simulink model "ROS2_simulink_UE5_0821"  (R2024b)
settings: Solver=VariableStepAuto  StartTime=0.0  StopTime=inf  RelTol=1e-3
undefined symbols (not defined in the file): Aw_pont, B_pont, Cb_pont, dt, Earth, I_L, I_T, IC, Ig_CG, k_neg, k_pos, L, l1, l2, LCF, m, rg, Sim3dSensor, T_yaw, trim_setpoint, Umax, WGS84, x, y, z
libraries: sim3dlib x12, ros2lib x8, matrix_library x8, sharedutil x7, uavsimlib x6, simulink x4, simulink_extras x4, sharedtransform x3, robotcorelib x1, aerolibtransform2 x1, sim3dcameralib x1, visionsinks x1
(part 1 of 2)
settings Model: Creator=qwv  LastModifiedBy=qwv

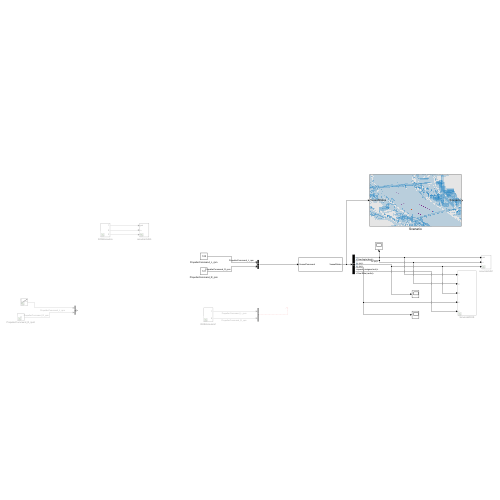
[thumbnail: Simulink's stored preview of the top-level diagram]
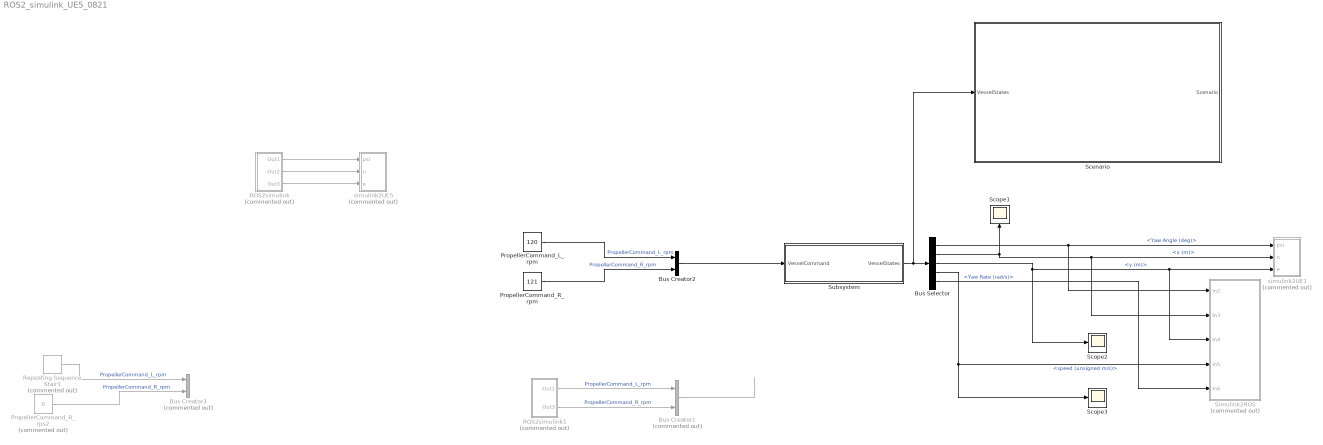
== system ROS2_simulink_UE5_0821 ==
  Bus Creator1 : BusCreator  Commented=on  Inputs=2
  Bus Creator2 : BusCreator  Inputs=3
  Bus Creator3 : BusCreator  Commented=on  Inputs=2
  Bus Selector : BusSelector  OutputSignals=Yaw Angle (deg),x (m),y (m),speed (unsigned m/s),Yaw Rate (rad/s)
  PropellerCommand_L_rpm : Constant  Value=120
  PropellerCommand_R_rpm : Constant  Value=121
  PropellerCommand_R_rps2 : Constant  Commented=on  Value=0
  ROS2simulink : Subsystem  Commented=on
  ROS2simulink1 : Subsystem  Commented=on
  Repeating Sequence Stair1 : simulink/Sources/Repeating Sequence Stair  Commented=on  OutValues=[-320 -300 -280 -260 -240 -220 -200 -180 -160 -140 -120 -100 -80 -60 -40 -20 0 20 40 60 80 100 120 140 160 180 200 220 240 260 280 300 320].'  tsamp=10  OutMin=[]  OutMax=[]  OutDataTypeStr=double  OutputDataTypeScalingMode=double  OutDataType=fixdt(0,8)  ConRadixGroup=Best Precision: Vector-wise  OutScaling=2^-12
  Scenario : Subsystem
      mask Display: image('ScenarioLondon.png'); % Use "Edit Image" on toolstrip to change.
  Scope1 : Scope
  Scope2 : Scope
  Scope3 : Scope
  Simulink2ROS : Subsystem  Commented=on
  Subsystem : Subsystem
  simulink2UE1 : Subsystem  Commented=on
  simulink2UE5 : Subsystem  Commented=on
  wires:
  ROS2simulink/1(Out1) -> simulink2UE5/1(psi)
  ROS2simulink/2(Out2) -> simulink2UE5/2(n)
  ROS2simulink/3(Out3) -> simulink2UE5/3(e)
  Bus Selector/3 -> Simulink2ROS/3(In4), simulink2UE1/3(e), Scope2/1  "<y (m)>"
  Bus Selector/2 -> Simulink2ROS/2(In3), simulink2UE1/2(n), Scope1/1  "<x (m)>"
  Subsystem/1(VesselStates) -> Scenario/1(VesselStates), Bus Selector/1
  Bus Selector/4 -> Scope3/1, Simulink2ROS/4(In5)  "<speed (unsigned m/s)>"
  Bus Selector/1 -> Simulink2ROS/1(In2), simulink2UE1/1(psi)  "<Yaw Angle (deg)>"
  ROS2simulink1/1(Out1) -> Bus Creator1/1  "PropellerCommand_L_rpm"
  ROS2simulink1/2(Out3) -> Bus Creator1/2  "PropellerCommand_R_rpm"
  Bus Selector/5 -> Simulink2ROS/5(In6)  "<Yaw Rate (rad/s)>"
  PropellerCommand_R_rpm/1 -> Bus Creator2/3  "PropellerCommand_R_rpm"
  PropellerCommand_L_rpm/1 -> Bus Creator2/1  "PropellerCommand_L_rpm"
  Bus Creator1/1 -> ?
  Bus Creator2/1 -> Subsystem/1(VesselCommand)
  Repeating Sequence Stair1/1 -> Bus Creator3/1  "PropellerCommand_L_rpm"
  PropellerCommand_R_rps2/1 -> Bus Creator3/2  "PropellerCommand_R_rpm"

== system ROS2_simulink_UE5_0821/ROS2simulink ==
  Blank Message : ros2lib/Blank Message  Commented=on  messageClass=Message  entityType=geometry_msgs/Point  messageType=geometry_msgs/Point  SampleTime=inf
  Bus Assignment : BusAssignment  Commented=on  AssignedSignals=x,z
  Bus Selector : BusSelector  OutputSignals=psi,n,e
  Bus Selector1 : BusSelector  Commented=on  OutputSignals=data
  Constant : Constant  Commented=on
  Constant1 : Constant  Commented=on
  Constant2 : Constant  Commented=on
  Display{,1..3} (4 alike) : Display
  Publish : ros2lib/Publish  Commented=on  topicSource=Specify your own  topic=/my_topic  messageType=geometry_msgs/Twist  QOSHistory=Keep last  QOSDepth=1  QOSReliability=Reliable  QOSDurability=Volatile  QOSDeadline=Inf  QOSLifespan=Inf  QOSLiveliness=Automatic  QOSLeaseDuration=Inf  QOSAvoidROSNamespaceConventions=off
  Sine Wave : Sin  Commented=on  SampleTime=0
  Sine Wave1 : Sin  Commented=on  SampleTime=0
  Subscribe : ros2lib/Subscribe  topicSource=Select from ROS network  topic=/topic_state  messageType=pid_interfaces/Command  sampleTime=-1  QOSHistory=Keep last  QOSDepth=1  QOSReliability=Reliable  QOSDurability=Volatile  QOSDeadline=Inf  QOSLifespan=Inf  QOSLiveliness=Automatic  QOSLeaseDuration=Inf  QOSAvoidROSNamespaceConventions=off
  Out1 : Outport
  Out2 : Outport  Port=2
  Out3 : Outport  Port=3
  wires:
  Bus Assignment/1 -> Publish/1
  Sine Wave1/1 -> Bus Assignment/3
  Blank Message/1 -> Bus Assignment/1
  Sine Wave/1 -> Bus Assignment/2
  Bus Selector/1 -> Out1/1, Display/1  "<psi>"
  Bus Selector/3 -> Out3/1, Display1/1  "<e>"
  Bus Selector/2 -> Display2/1, Out2/1  "<n>"
  Bus Selector1/1 -> Display3/1  "<data>"
  Subscribe/2 -> Bus Selector/1

== system ROS2_simulink_UE5_0821/ROS2simulink1 ==
  Bus Selector : BusSelector  OutputSignals=rpm_e_l,rpm_e_r
  Data Type Conversion : DataTypeConversion  SaturateOnIntegerOverflow=off  RndMeth=Floor
  Data Type Conversion1 : DataTypeConversion  SaturateOnIntegerOverflow=off  RndMeth=Floor
  Display1 : Display
  Display2 : Display
  Subscribe : ros2lib/Subscribe  topicSource=Select from ROS network  topic=/topic_state  messageType=pid_interfaces/Command  sampleTime=-1  QOSHistory=Keep last  QOSDepth=1  QOSReliability=Reliable  QOSDurability=Volatile  QOSDeadline=Inf  QOSLifespan=Inf  QOSLiveliness=Automatic  QOSLeaseDuration=Inf  QOSAvoidROSNamespaceConventions=off
  Out1 : Outport
  Out3 : Outport  Port=2
  wires:
  Bus Selector/2 -> Display1/1, Data Type Conversion1/1  "<rpm_e_r>"
  Subscribe/2 -> Bus Selector/1
  Data Type Conversion/1 -> Out1/1
  Data Type Conversion1/1 -> Out3/1
  Bus Selector/1 -> Data Type Conversion/1, Display2/1  "<rpm_e_l>"

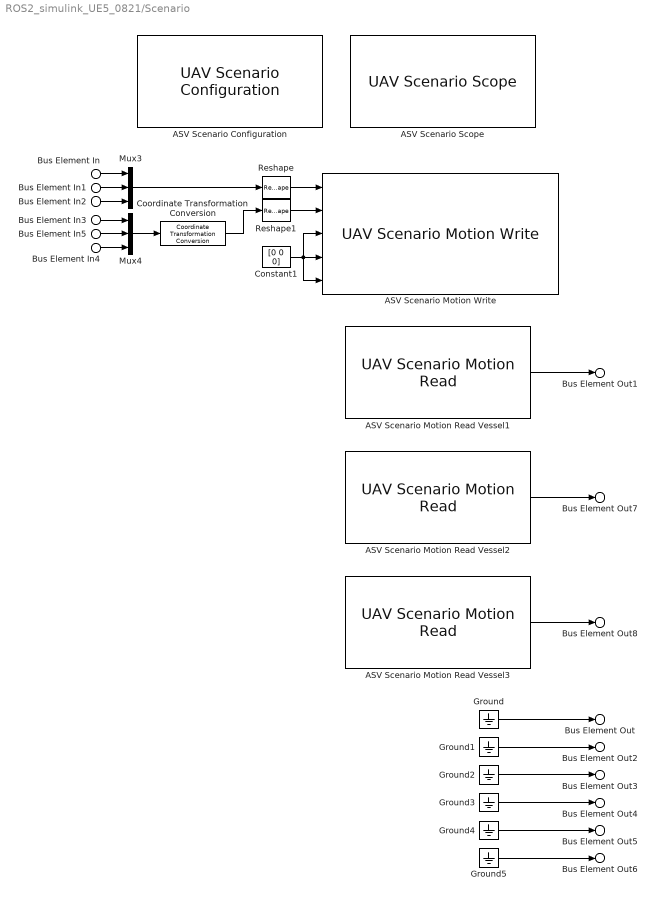
== system ROS2_simulink_UE5_0821/Scenario ==
  Bus Element In : Inport  PortName=VesselStates  Element=x (m)
  Bus Element In1 : Inport  PortName=VesselStates  Element=y (m)
  Bus Element In2 : Inport  PortName=VesselStates  Element=z (m)
  Bus Element In3 : Inport  PortName=VesselStates  Element=Yaw Angle (rad)
  Bus Element In4 : Inport  PortName=VesselStates  Element=Roll Angle (rad)
  Bus Element In5 : Inport  PortName=VesselStates  Element=Pitch Angle (rad)
  ASV Scenario Configuration : uavsimlib/UAV Scenario Configuration  Priority=-1  UAVScenarioObject=Scenario  SampleTime=dt.cuboid  UpdateParam=false  SensorMotionBusName='SensorMotionBus'  PlatformMotionBusName='PlatformMotionBus'  ScenarioMotionBusName='ScenarioMotionBus'  ScenarioMotionSignalName='ScenarioMotions'
      settings: AttributesFormatString=%<UAVScenarioObject>
  ASV Scenario Motion Read Vessel1 : uavsimlib/UAV Scenario Motion Read  Priority=1  EntityName='Vessel1Yacht'  ReferenceFrame=NED  OutputWind=off
      settings: AttributesFormatString=%<EntityName>
  ASV Scenario Motion Read Vessel2 : uavsimlib/UAV Scenario Motion Read  Priority=1  EntityName='Vessel2RegularBoat'  ReferenceFrame=NED  OutputWind=off
      settings: AttributesFormatString=%<EntityName>
  ASV Scenario Motion Read Vessel3 : uavsimlib/UAV Scenario Motion Read  Priority=1  EntityName='Vessel3Sailboat'  ReferenceFrame=NED  OutputWind=off
      settings: AttributesFormatString=%<EntityName>
  ASV Scenario Motion Write : uavsimlib/UAV Scenario Motion Write  Priority=0  PlatName='EgoVessel'  ReferenceFrame=NED
      settings: AttributesFormatString=%<PlatName>
  "ASV Scenario Scope " : uavsimlib/UAV Scenario Scope  Priority=1  SensorNameTable={}  SampleTime=dt.cuboid
  Constant1 : Constant  Value=[0 0 0]
  Coordinate Transformation Conversion : robotcorelib/Coordinate Transformation Conversion  InputRepresentation=Euler Angles  InputEulerSequence=ZYX  ShowTrVecInputPort=on  OutputRepresentation=Quaternion  OutputEulerSequence=ZYX  ShowTrVecOutputPort=on  SimulateUsing=Interpreted execution
  Ground{,1..5} (6 alike) : Ground
  Mux3 : Mux  Inputs=3
  Mux4 : Mux  Inputs=3
  Reshape : Reshape  OutputDimensionality=Customize  OutputDimensions=[1,3]
  Reshape1 : Reshape  OutputDimensionality=Customize  OutputDimensions=[1,4]
  Bus Element Out1 : Outport  PortName=Scenario  Element=Vessel1.Motion
  Bus Element Out : Outport  PortName=Scenario  Element=EgoVessel.Lidar
  Bus Element Out2 : Outport  PortName=Scenario  Element=EgoVessel.Radar
  Bus Element Out3 : Outport  PortName=Scenario  Element=EgoVessel.Camera.Front
  Bus Element Out4 : Outport  PortName=Scenario  Element=EgoVessel.Camera.Back
  Bus Element Out5 : Outport  PortName=Scenario  Element=EgoVessel.Camera.Starboard
  Bus Element Out6 : Outport  PortName=Scenario  Element=EgoVessel.Camera.Port
  Bus Element Out7 : Outport  PortName=Scenario  Element=Vessel2.Motion
  Bus Element Out8 : Outport  PortName=Scenario  Element=Vessel3.Motion
  wires:
  Bus Element In/1 -> Mux3/1
  Coordinate Transformation Conversion/1 -> Reshape1/1
  Bus Element In2/1 -> Mux3/3
  Bus Element In1/1 -> Mux3/2
  Mux4/1 -> Coordinate Transformation Conversion/1
  Reshape/1 -> ASV Scenario Motion Write/1
  Mux3/1 -> Reshape/1
  Bus Element In3/1 -> Mux4/1
  Reshape1/1 -> ASV Scenario Motion Write/2
  Constant1/1 -> ASV Scenario Motion Write/5, ASV Scenario Motion Write/4, ASV Scenario Motion Write/3
  Ground/1 -> Bus Element Out/1
  Ground1/1 -> Bus Element Out2/1
  Ground2/1 -> Bus Element Out3/1
  Ground3/1 -> Bus Element Out4/1
  Ground4/1 -> Bus Element Out5/1
  Ground5/1 -> Bus Element Out6/1
  Bus Element In5/1 -> Mux4/2
  Bus Element In4/1 -> Mux4/3
  ASV Scenario Motion Read Vessel1/1 -> Bus Element Out1/1
  ASV Scenario Motion Read Vessel2/1 -> Bus Element Out7/1
  ASV Scenario Motion Read Vessel3/1 -> Bus Element Out8/1

== system ROS2_simulink_UE5_0821/Simulink2ROS ==
  In2 : Inport
  In3 : Inport  Port=2
  In4 : Inport  Port=3
  In5 : Inport  Port=4
  In6 : Inport  Port=5
  Blank Message : ros2lib/Blank Message  messageClass=Message  entityType=geometry_msgs/Point  messageType=geometry_msgs/Point  SampleTime=-1
  Blank Message1 : ros2lib/Blank Message  messageClass=Message  entityType=geometry_msgs/Point  messageType=geometry_msgs/Point  SampleTime=-1
  Bus Assignment : BusAssignment  AssignedSignals=z,x,y
  Bus Assignment1 : BusAssignment  AssignedSignals=x,y
  Publish : ros2lib/Publish  topicSource=Specify your own  topic=/usvState_from_matlab  messageType=geometry_msgs/Point  QOSHistory=Keep last  QOSDepth=1  QOSReliability=Reliable  QOSDurability=Volatile  QOSDeadline=Inf  QOSLifespan=Inf  QOSLiveliness=Automatic  QOSLeaseDuration=Inf  QOSAvoidROSNamespaceConventions=off
  Publish1 : ros2lib/Publish  topicSource=Specify your own  topic=/usvVel_from_matlab  messageType=geometry_msgs/Point  QOSHistory=Keep last  QOSDepth=1  QOSReliability=Reliable  QOSDurability=Volatile  QOSDeadline=Inf  QOSLifespan=Inf  QOSLiveliness=Automatic  QOSLeaseDuration=Inf  QOSAvoidROSNamespaceConventions=off
  Sine Wave : Sin  Commented=on  Phase=-pi/2  SampleTime=0.01
  Sine Wave1 : Sin  Commented=on  SampleTime=0.01
  wires:
  Bus Assignment/1 -> Publish/1
  Blank Message/1 -> Bus Assignment/1
  In3/1 -> Bus Assignment/3  "x"
  In2/1 -> Bus Assignment/2  "yaw"
  In4/1 -> Bus Assignment/4  "y"
  In5/1 -> Bus Assignment1/2  "x"
  In6/1 -> Bus Assignment1/3  "y"
  Blank Message1/1 -> Bus Assignment1/1
  Bus Assignment1/1 -> Publish1/1

== system ROS2_simulink_UE5_0821/Subsystem ==
  VesselCommand : Inport
  "Environment                      " : Subsystem
      settings: PortSchema="{\"entries\":[{\"content\":{\"sides\":[{\"content\":{\"connectorIds\":[]},\"type\":\"ConnectorPlacement.EquallySpacedRectSide\",\"uuid\":\"fca19152-fc00-4d56-ba92-14fe63ef36b4\"},{\"content\":{\"connectorIds\":[],\"side\":\"RIGHT\"},\"type\":\"ConnectorPlacement.EquallySpacedRectSide\",\"uuid\":\"9b72ab77-7e08-482e-83b0-310cce3c8f1a\"},{\"content\":{\"connectorIds\":[],\"side\":\"TOP\"},\"type\":\"ConnectorPlacement.EquallySpacedRectSide\",\"uuid\":\"75056a42-0ec0-4a62-a716-716d3d08c743\"},{\"content\":{\"connectorIds\":[\"Out1\"],\"side\":\"BOTTOM\"},\"type\":\"ConnectorPlacement.EquallySpacedRectSide\",\"uuid\":\"a83eb91f-f17a-4b40-9f51-3dae26c6d747\"}]},\"type\":\"ConnectorPlacement.EquallySpacedConnector\",\"uuid\":\"95b30908-6da5-4486-944b-c5a247aaa1bb\"}],\"packageUris\":[\"http://schema.mathworks.com/mf0/Connector/R2020b\"],\"version\":\"1.0\"}"
      mask Display: image('wave.png'); % Use "Edit Image" on toolstrip to change.
  "Payload               " : Subsystem
      settings: PortSchema="{\"entries\":[{\"content\":{\"sides\":[{\"content\":{\"connectorIds\":[]},\"type\":\"ConnectorPlacement.EquallySpacedRectSide\",\"uuid\":\"fca19152-fc00-4d56-ba92-14fe63ef36b4\"},{\"content\":{\"connectorIds\":[],\"side\":\"RIGHT\"},\"type\":\"ConnectorPlacement.EquallySpacedRectSide\",\"uuid\":\"9b72ab77-7e08-482e-83b0-310cce3c8f1a\"},{\"content\":{\"connectorIds\":[],\"side\":\"TOP\"},\"type\":\"ConnectorPlacement.EquallySpacedRectSide\",\"uuid\":\"75056a42-0ec0-4a62-a716-716d3d08c743\"},{\"content\":{\"connectorIds\":[\"Out1\"],\"side\":\"BOTTOM\"},\"type\":\"ConnectorPlacement.EquallySpacedRectSide\",\"uuid\":\"de76c6b2-9f00-4f8e-b9aa-5205882fe021\"}]},\"type\":\"ConnectorPlacement.EquallySpacedConnector\",\"uuid\":\"95b30908-6da5-4486-944b-c5a247aaa1bb\"}],\"packageUris\":[\"http://schema.mathworks.com/mf0/Connector/R2020b\"],\"version\":\"1.0\"}"
      mask Display: image('Payload.png'); % Use "Edit Image" on toolstrip to change.
  Vessel Platform : Subsystem
      settings: PortSchema="{\"entries\":[{\"content\":{\"sides\":[{\"content\":{\"connectorIds\":[\"In1\"]},\"type\":\"ConnectorPlacement.EquallySpacedRectSide\",\"uuid\":\"07d72031-313d-4f7a-8748-a204c86c4fb3\"},{\"content\":{\"connectorIds\":[\"Out1\"],\"side\":\"RIGHT\"},\"type\":\"ConnectorPlacement.EquallySpacedRectSide\",\"uuid\":\"44ee2045-6692-4365-9cdf-18d58720c318\"},{\"content\":{\"connectorIds\":[\"In2\",\"In3\"],\"side\":\"TOP\"},\"type\":\"ConnectorPlacement.EquallySpacedRectSide\",\"uuid\":\"f88d81e2-ba48-4dce-adbc-b28d38415594\"}]},\"type\":\"ConnectorPlacement.EquallySpacedConnector\",\"uuid\":\"d3df33cd-3b96-4401-b0f4-089d5266b772\"}],\"packageUris\":[\"http://schema.mathworks.com/mf0/Connector/R2020b\"],\"version\":\"1.0\"}"
      mask Display: image('VesselPlatform.png'); % Use "Edit Image" on toolstrip to change.
  VesselStates : Outport
  wires:
  "Payload               "/1(Payload) -> Vessel Platform/2(Payload)
  Vessel Platform/1(VesselStates) -> VesselStates/1
  "Environment                      "/1(Environment) -> Vessel Platform/3(Environment)
  VesselCommand/1 -> Vessel Platform/1(VesselCommand)

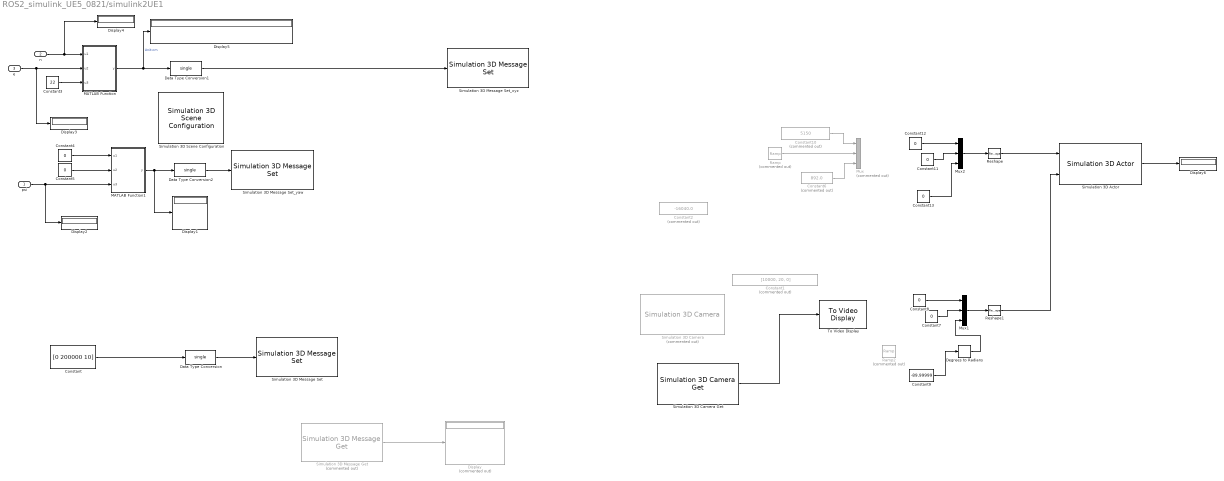
== system ROS2_simulink_UE5_0821/simulink2UE1 ==
  psi : Inport
  n : Inport  Port=2
  e : Inport  Port=3
  Constant : Constant  Value=[0 200000 10]  VectorParams1D=off  OutDataTypeStr=single
  Constant1 : Constant  Commented=on  Value=[10000, 20, 0]  VectorParams1D=off
  Constant10 : Constant  Commented=on  Value=5150
  Constant{4..5,7..8,11..13} (7 alike) : Constant  Value=0
  Constant2 : Constant  Commented=on  Value=-16040.0
  Constant3 : Constant  Value=22
  Constant6 : Constant  Commented=on  Value=892.0
  Constant9 : Constant  Value=-89.99999
  Data Type Conversion : DataTypeConversion  OutDataTypeStr=single  SaturateOnIntegerOverflow=off  RndMeth=Floor
  Data Type Conversion1 : DataTypeConversion  OutDataTypeStr=single  SaturateOnIntegerOverflow=off  RndMeth=Floor
  Data Type Conversion2 : DataTypeConversion  OutDataTypeStr=single  SaturateOnIntegerOverflow=off  RndMeth=Floor
  Degrees to Radians : simulink_extras/Transformations/Degrees to Radians
  Display : Display  Commented=on
  Display{1..6} (6 alike) : Display
  MATLAB Function : MATLAB Function  TreatAsAtomicUnit=on
  MATLAB Function1 : MATLAB Function  TreatAsAtomicUnit=on
  Mux : Mux  Commented=on  Inputs=3
  Mux1 : Mux  Inputs=3
  Mux2 : Mux  Inputs=3
  Ramp : simulink/Sources/Ramp  Commented=on  slope=-1000  start=0  InitialOutput=-16040.0
  Ramp2 : simulink/Sources/Ramp  Commented=on  slope=10  start=0  InitialOutput=0
  Reshape : Reshape  OutputDimensionality=Customize  OutputDimensions=[1,3]
  Reshape1 : Reshape  OutputDimensionality=Customize  OutputDimensions=[1,3]
  Simulation 3D Actor : sim3dlib/Simulation 3D Actor  Priority=1  ActorName=cxzCamera  ParentName=Scene Origin  Operation=Create at setup  InitScriptText=|  SampleTime=-1  Translation=[0 0 0]  Rotation=[0 0 0]  Scale=[1 1 1]  InputsText=cxzCamera.Translation cxzCamera.Rotation  aMode=5  ActorTag=cxzCamera  ActorType=Sim3dActor  ID=C
      | % Reserved keywords:
      | % - Actor : handle to this actor object
      | % - World : handle to the world object
      | 
      | % Examples:
      | 
      | % Create a primitive geometry (optional)
      | % createShape(Actor, 'box', [1 1 1]);
      | 
      | % Initialize values (optional)
      | % Actor.Physics = true;
      | % Actor.Color = [1 0 0];
  Simulation 3D Camera : sim3dcameralib/Simulation 3D Camera  Priority=1  Commented=on  sensorTag=Sim3dSensor�  sensorId=3  sensorName=Sim3dSensor�  vehTagList={'Scene Origin';'cxzCamera'}  vehTag=cxzCamera  mountLoc=Origin  offsetFlag=off  tmountOffset=[100, 100, 0]  extTmount=off  rmountOffset=[0, 0, 0]  extRmount=off  FocalLength=[1109, 1109]  OpticalCenter=[640, 360]  ImageSize=[720, 1280]  RadialDistortion=[0, 0]  TangentialDistortion=[0, 0]  SensorSkew=0  DepthOutportEnabled=off  SemanticOutportEnabled=off  TransformOutportEnabled=off  SampleTime=-1  mountPoint=[0 0 0]  mountOrientation=[0 0 0]  aMode=3  ID=3
      settings: LibrarySourceBlock=drivingsim3d/Simulation 3D Camera
  Simulation 3D Camera Get : sim3dlib/Simulation 3D Camera Get  Priority=1  sensorTag=Sim3dSensor�  sensorId=1  sensorName=Sim3dSensor�  vehTagList={'Scene Origin';'cxzCamera'}  vehTag=cxzCamera  mountLoc=Origin  offsetFlag=off  tmountOffset=[0, 0, 0]  rmountOffset=[0, 0, 0]  HorizontalResolution=1920  VerticalResolution=1080  HorizontalFOV=90  SampleTime=-1  mountPoint=[0 0 0]  mountOrientation=[0 0 0]  aMode=5  ID=1
      settings: LibrarySourceBlock=sl3dlib/Simulation 3D/Utilities/Simulation 3D Camera Get
  Simulation 3D Message Get : sim3dlib/Simulation 3D Message Get  Priority=1  Commented=on  SigName=boatGet  DataType=single  MsgSize=[1 3]  Ts=-1  aMode=2
      settings: LibrarySourceBlock=vehdynlibsim3dcore/Simulation 3D Message Get
  Simulation 3D Message Set : sim3dlib/Simulation 3D Message Set  Priority=-1  SigName=boatSet  Ts=-1  aMode=2
      settings: LibrarySourceBlock=vehdynlibsim3dcore/Simulation 3D Message Set
  Simulation 3D Message Set_xyz : sim3dlib/Simulation 3D Message Set  Priority=-1  SigName=boatSet_xyz  Ts=-1  aMode=2
      settings: LibrarySourceBlock=vehdynlibsim3dcore/Simulation 3D Message Set
  Simulation 3D Message Set_yaw : sim3dlib/Simulation 3D Message Set  Priority=-1  SigName=boatSet_yaw  Ts=-1  aMode=2
      settings: LibrarySourceBlock=vehdynlibsim3dcore/Simulation 3D Message Set
  Simulation 3D Scene Configuration : sim3dlib/Simulation 3D Scene Configuration  Priority=0  ProjectFormat=Unreal Editor  SceneDesc=Straight road  ProjectName=F:\MATLAB2024b\toolbox\shared\sim3d_projects\automotive_project_windows\UE\WindowsNoEditor\VehicleSimulation.exe  ScenePath=/Game/Maps/HwStrght  UEProjPath=D:\UE5_myPrograms\ProjectUE5.3\TestSim3dGetSet\TestSim3dGetSet.uproject  EnableOpenDRIVE=off  vehTagList={'Custom';'Scene Origin';'cxzCamera'}  vehTag=Scene Origin  FreeCameraInitialTranslation=[0, 0, 0]  FreeCameraDefaultInitialTranslation=[-6, 0, 2]  FreeCameraInitialRotation=[0, 0, 0]  FreeCameraDefaultInitialRotation=[0, -15, 0]  OpVisEn=off  Ts=0.02  EnableWindow=on  EnableRemoteAccess=off  EnableWeather=off  SunAzimuth=90  SunAltitude=40.0  EnableGeospatialSun=off  Latitude=0  Longitude=0  Date=2023-01-01  Time=10:30:00  GeoTimeZone=-5.0  SunDaylightSaving=off  wind=1  clouds=10  EnableVolumetricClouds=off  CloudCoverage=0  CloudAltitude=6  fog=0  rain=0  RaindropsEffect=off  SnowDensity=0  EnableGeospatial=off  UseTrueOrigin=off  OriginHeight=200  OriginLatitude=40.744652  OriginLongitude=-73.988864  MapStyle=Aerial  AdditionalAssetIDs=[]  UseAdvancedSunSky=off  SolarTime=11  TimeZone=-5  Day=21  Month=9  Year=2022  UseDaylightSavingTime=on  DSTStartDay=10  DSTStartMonth=3  DSTEndDay=3  DSTEndMonth=11  DSTSwitchHour=2  sensorTag=MainCamera2  sensorId=2  sensorName=MainCamera2  mountLoc=Origin  offsetFlag=off  tmountOffset=[0, 0, 0]  rmountOffset=[0, 0, 0]  HorizontalResolution=1280  VerticalResolution=720  HorizontalFOV=60  mountPoint=[0 0 0]  mountOrientation=[0 0 0]  aMode=2  ID=2  GeoTrigger=Inactive
      settings: LibrarySourceBlock=vehdynlibsim3dcore/Simulation 3D Scene Configuration
  To Video Display : visionsinks/To Video Display  windowSizeMode=Normal  openAtMdlStart=on  fullScreen=off  videoWindowX=752  videoWindowY=227  saveWindowSize=off  videoWindowWidth=1280  videoWindowHeight=720  inputColorFormat=RGB  inputType=Obsolete  imagePorts=One multidimensional signal  OutputDevice=On-screen video monitor  dataOrg=Column-major  isWindowOpen=off
  wires:
  Simulation 3D Message Get/1 -> Display/1
  Data Type Conversion/1 -> Simulation 3D Message Set/1
  Constant/1 -> Data Type Conversion/1
  Data Type Conversion1/1 -> Simulation 3D Message Set_xyz/1
  Data Type Conversion2/1 -> Simulation 3D Message Set_yaw/1
  psi/1 -> Display2/1, MATLAB Function1/3(u3)
  e/1 -> MATLAB Function/2(u2), Display3/1
  n/1 -> Display4/1, MATLAB Function/1(u1)
  Constant3/1 -> MATLAB Function/3(u3)
  MATLAB Function/1(y) -> Data Type Conversion1/1, Display5/1  "Unit:cm"
  Constant4/1 -> MATLAB Function1/1(u1)
  Constant5/1 -> MATLAB Function1/2(u2)
  MATLAB Function1/1(y) -> Display1/1, Data Type Conversion2/1
  Simulation 3D Actor/1 -> Display6/1
  Constant7/1 -> Mux1/2
  Degrees to Radians/1 -> Mux1/3
  Constant8/1 -> Mux1/1
  Constant6/1 -> Mux/3
  Mux1/1 -> Reshape1/1
  Reshape1/1 -> Simulation 3D Actor/2
  Reshape/1 -> Simulation 3D Actor/1
  Constant10/1 -> Mux/1
  Ramp/1 -> Mux/2
  Simulation 3D Camera Get/1 -> To Video Display/1
  Constant9/1 -> Degrees to Radians/1
  Constant11/1 -> Mux2/2
  Constant12/1 -> Mux2/1
  Constant13/1 -> Mux2/3
  Mux2/1 -> Reshape/1

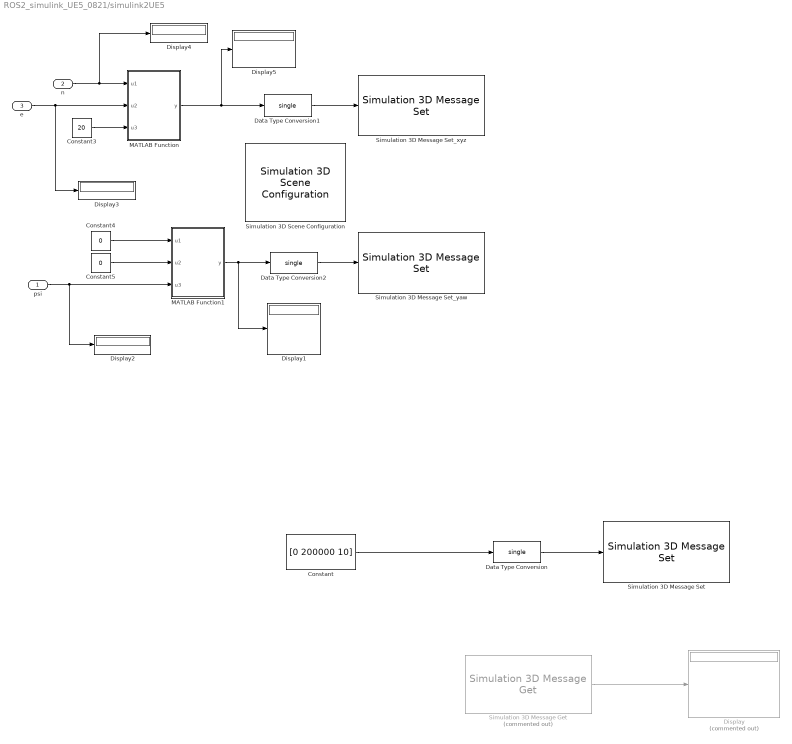
== system ROS2_simulink_UE5_0821/simulink2UE5 ==
  psi : Inport
  n : Inport  Port=2
  e : Inport  Port=3
  Constant : Constant  Value=[0 200000 10]  VectorParams1D=off  OutDataTypeStr=single
  Constant3 : Constant  Value=20
  Constant4 : Constant  Value=0
  Constant5 : Constant  Value=0
  Data Type Conversion : DataTypeConversion  OutDataTypeStr=single  SaturateOnIntegerOverflow=off  RndMeth=Floor
  Data Type Conversion1 : DataTypeConversion  OutDataTypeStr=single  SaturateOnIntegerOverflow=off  RndMeth=Floor
  Data Type Conversion2 : DataTypeConversion  OutDataTypeStr=single  SaturateOnIntegerOverflow=off  RndMeth=Floor
  Display : Display  Commented=on
  Display{1..5} (5 alike) : Display
  MATLAB Function : MATLAB Function  TreatAsAtomicUnit=on
  MATLAB Function1 : MATLAB Function  TreatAsAtomicUnit=on
  Simulation 3D Message Get : sim3dlib/Simulation 3D Message Get  Priority=1  Commented=on  SigName=boatGet  DataType=single  MsgSize=[1 3]  Ts=-1  aMode=2
      settings: LibrarySourceBlock=vehdynlibsim3dcore/Simulation 3D Message Get
  Simulation 3D Message Set : sim3dlib/Simulation 3D Message Set  Priority=-1  SigName=boatSet  Ts=-1  aMode=2
      settings: LibrarySourceBlock=vehdynlibsim3dcore/Simulation 3D Message Set
  Simulation 3D Message Set_xyz : sim3dlib/Simulation 3D Message Set  Priority=-1  SigName=boatSet_xyz  Ts=-1  aMode=2
      settings: LibrarySourceBlock=vehdynlibsim3dcore/Simulation 3D Message Set
  Simulation 3D Message Set_yaw : sim3dlib/Simulation 3D Message Set  Priority=-1  SigName=boatSet_yaw  Ts=-1  aMode=2
      settings: LibrarySourceBlock=vehdynlibsim3dcore/Simulation 3D Message Set
  Simulation 3D Scene Configuration : sim3dlib/Simulation 3D Scene Configuration  Priority=0  ProjectFormat=Unreal Editor  SceneDesc=Straight road  ProjectName=F:\MATLAB2024b\toolbox\shared\sim3d_projects\automotive_project_windows\UE\WindowsNoEditor\VehicleSimulation.exe  ScenePath=/Game/Maps/HwStrght  UEProjPath=D:\UE5_myPrograms\ProjectUE5.3\TestSim3dGetSet\TestSim3dGetSet.uproject  EnableOpenDRIVE=off  vehTagList={'Custom';'Scene Origin'}  vehTag=Scene Origin  FreeCameraInitialTranslation=[0, 0, 0]  FreeCameraDefaultInitialTranslation=[-6, 0, 2]  FreeCameraInitialRotation=[0, 0, 0]  FreeCameraDefaultInitialRotation=[0, -15, 0]  OpVisEn=off  Ts=.02  EnableWindow=on  EnableRemoteAccess=off  EnableWeather=off  SunAzimuth=90  SunAltitude=40.0  EnableGeospatialSun=off  Latitude=0  Longitude=0  Date=2023-01-01  Time=10:30:00  GeoTimeZone=-5.0  SunDaylightSaving=off  wind=1  clouds=10  EnableVolumetricClouds=off  CloudCoverage=0  CloudAltitude=6  fog=0  rain=0  RaindropsEffect=off  SnowDensity=0  EnableGeospatial=off  UseTrueOrigin=off  OriginHeight=200  OriginLatitude=40.744652  OriginLongitude=-73.988864  MapStyle=Aerial  AdditionalAssetIDs=[]  UseAdvancedSunSky=off  SolarTime=11  TimeZone=-5  Day=21  Month=9  Year=2022  UseDaylightSavingTime=on  DSTStartDay=10  DSTStartMonth=3  DSTEndDay=3  DSTEndMonth=11  DSTSwitchHour=2  sensorTag=MainCamera1  sensorId=1  sensorName=MainCamera1  mountLoc=Origin  offsetFlag=off  tmountOffset=[0, 0, 0]  rmountOffset=[0, 0, 0]  HorizontalResolution=1280  VerticalResolution=720  HorizontalFOV=60  mountPoint=[0 0 0]  mountOrientation=[0 0 0]  aMode=2  ID=1  GeoTrigger=Inactive
      settings: LibrarySourceBlock=vehdynlibsim3dcore/Simulation 3D Scene Configuration
  wires:
  Simulation 3D Message Get/1 -> Display/1
  Data Type Conversion/1 -> Simulation 3D Message Set/1
  Constant/1 -> Data Type Conversion/1
  Data Type Conversion1/1 -> Simulation 3D Message Set_xyz/1
  Data Type Conversion2/1 -> Simulation 3D Message Set_yaw/1
  psi/1 -> Display2/1, MATLAB Function1/3(u3)
  e/1 -> MATLAB Function/2(u2), Display3/1
  n/1 -> Display4/1, MATLAB Function/1(u1)
  Constant3/1 -> MATLAB Function/3(u3)
  MATLAB Function/1(y) -> Data Type Conversion1/1, Display5/1
  Constant4/1 -> MATLAB Function1/1(u1)
  Constant5/1 -> MATLAB Function1/2(u2)
  MATLAB Function1/1(y) -> Display1/1, Data Type Conversion2/1

== system ROS2_simulink_UE5_0821/Subsystem/Environment                       ==
  note: T. I. Fossen and T. Perez (2004). Marine Systems Simulator (MSS). URL: https://github.com/cybergalactic/MSS
  Current : Subsystem
  Earth : Subsystem
  Water : Subsystem
  Bus Element Out : Outport  PortName=Environment  Element=Current
  Bus Element Out1 : Outport  PortName=Environment  Element=Water
  Bus Element Out2 : Outport  PortName=Environment  Element=Earth
  wires:
  Current/1(Current) -> Bus Element Out/1
  Earth/1(Earth) -> Bus Element Out2/1
  Water/1(Water) -> Bus Element Out1/1

== system ROS2_simulink_UE5_0821/Subsystem/Payload                ==
  note: T. I. Fossen and T. Perez (2004). Marine Systems Simulator (MSS). URL: https://github.com/cybergalactic/MSS
  Location of payload (m) : Constant  Value=[0 0 -0.35]
  Payload mass (kg) : Constant  Value=25
  Bus Element Out : Outport  PortName=Payload  Element=Payload mass (kg)
  Bus Element Out1 : Outport  PortName=Payload  Element=Location of payload (m)
  wires:
  Payload mass (kg)/1 -> Bus Element Out/1
  Location of payload (m)/1 -> Bus Element Out1/1

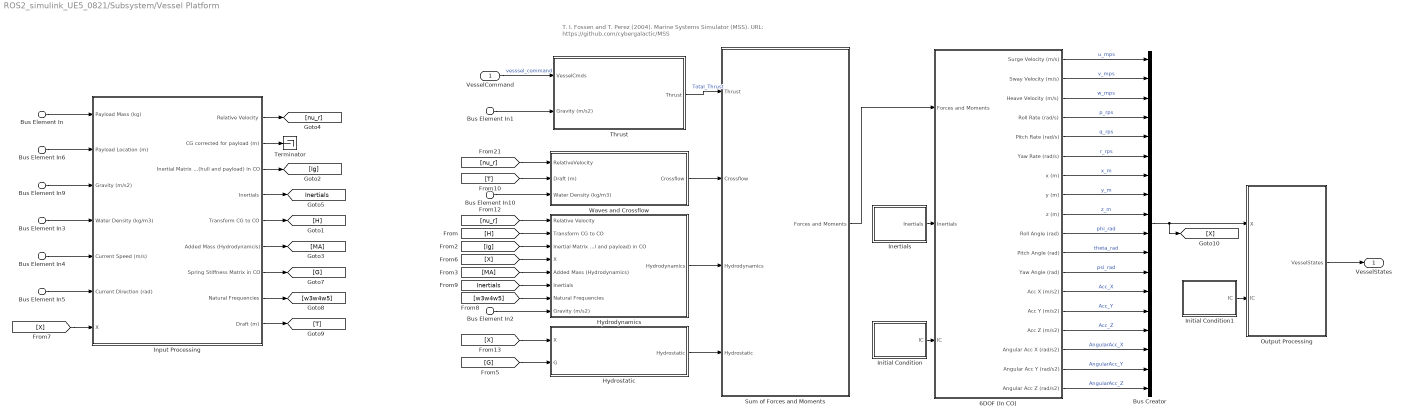
== system ROS2_simulink_UE5_0821/Subsystem/Vessel Platform ==
  note: T. I. Fossen and T. Perez (2004). Marine Systems Simulator (MSS). URL: https://github.com/cybergalactic/MSS
  VesselCommand : Inport
  Bus Element In : Inport  Port=2  PortName=Payload  Element=Payload mass (kg)
  Bus Element In6 : Inport  Port=2  PortName=Payload  Element=Location of payload (m)
  Bus Element In9 : Inport  Port=3  PortName=Environment  Element=Earth.Gravity (m/s2)
  Bus Element In2 : Inport  Port=3  PortName=Environment  Element=Earth.Gravity (m/s2)
  Bus Element In1 : Inport  Port=3  PortName=Environment  Element=Earth.Gravity (m/s2)
  Bus Element In3 : Inport  Port=3  PortName=Environment  Element=Water.Water Density (kg/m3)
  Bus Element In10 : Inport  Port=3  PortName=Environment  Element=Water.Water Density (kg/m3)
  Bus Element In4 : Inport  Port=3  PortName=Environment  Element=Current.Current speed (m/s)
  Bus Element In5 : Inport  Port=3  PortName=Environment  Element=Current.Current direction (rad)
  6DOF (In CO) : Subsystem
      mask Display: image('6DOF.png'); % Use "Edit Image" on toolstrip to change.
  Bus Creator : BusCreator  Inputs=18
  Hydrodynamics : Subsystem
      mask Display: image('Hydrodynamcis.png'); % Use "Edit Image" on toolstrip to change.
  Hydrostatic : Subsystem
      mask Display: image('Hydrostatic.png'); % Use "Edit Image" on toolstrip to change.
  Inertials : Subsystem
      mask Display: disp('Inertials');
  Initial Condition : Subsystem
      mask Display: disp('Initial Conditions');
  Initial Condition1 : Subsystem
  Input Processing : Subsystem
  Output Processing : Subsystem
  Sum of Forces and Moments : Subsystem
      mask Display: image('ForceAndMoment.png'); % Use "Edit Image" on toolstrip to change.
  Terminator : Terminator
  Thrust : Subsystem
      mask Display: image('propellerTwo.png'); % Use "Edit Image" on toolstrip to change.
  Waves and Crossflow : Subsystem
      mask Display: image('waves.png'); % Use "Edit Image" on toolstrip to change.
  VesselStates : Outport
  tag scope: Inertials=global
  wires:
  Thrust/1(Thrust) -> Sum of Forces and Moments/1(Thrust)  "Total_Thrust"
  [nu_r] -> Waves and Crossflow/1(RelativeVelocity)
  Bus Element In5/1 -> Input Processing/6(Current Direction (rad))
  6DOF (In CO)/1(Surge Velocity (m/s)) -> Bus Creator/1  "u_mps"
  6DOF (In CO)/2(Sway Velocity (m/s)) -> Bus Creator/2  "v_mps"
  6DOF (In CO)/3(Heave Velocity (m/s)) -> Bus Creator/3  "w_mps"
  6DOF (In CO)/4(Roll Rate (rad/s)) -> Bus Creator/4  "p_rps"
  6DOF (In CO)/5(Pitch Rate (rad/s)) -> Bus Creator/5  "q_rps"
  6DOF (In CO)/6(Yaw Rate (rad/s)) -> Bus Creator/6  "r_rps"
  6DOF (In CO)/7(x (m)) -> Bus Creator/7  "x_m"
  6DOF (In CO)/8(y (m)) -> Bus Creator/8  "y_m"
  6DOF (In CO)/9(z (m)) -> Bus Creator/9  "z_m"
  6DOF (In CO)/10(Roll Angle (rad)) -> Bus Creator/10  "phi_rad"
  6DOF (In CO)/11(Pitch Angle (rad)) -> Bus Creator/11  "theta_rad"
  6DOF (In CO)/12(Yaw Angle (rad)) -> Bus Creator/12  "psi_rad"
  Bus Creator/1 -> [X], Output Processing/1(X)
  [X] -> Hydrostatic/1(X)
  Sum of Forces and Moments/1(Forces and Moments) -> 6DOF (In CO)/1(Forces and Moments)
  Waves and Crossflow/1(Crossflow) -> Sum of Forces and Moments/2(Crossflow)
  Input Processing/6(Added Mass (Hydrodynamcis)) -> [MA]
  VesselCommand/1 -> Thrust/1(VesselCmds)  "vesssel_command"
  Bus Element In9/1 -> Input Processing/3(Gravity (m/s2))
  Bus Element In3/1 -> Input Processing/4(Water Density (kg/m3))
  Input Processing/5(Transform CG to CO) -> [H]
  Input Processing/3(Inertial Matrix (hull and payload) in CO) -> [Ig]
  Input Processing/1(Relative Velocity) -> [nu_r]
  [X] -> Input Processing/7(X)
  Input Processing/4(Inertials) -> [Inertials]
  Input Processing/7(Spring Stiffness Matrix in CO) -> [G]
  [G] -> Hydrostatic/2(G)
  Input Processing/8(Natural Frequencies) -> [w3w4w5]
  Bus Element In10/1 -> Waves and Crossflow/3("Water Density (kg/m3) ")
  Input Processing/9(Draft (m)) -> [T]
  [T] -> Waves and Crossflow/2(Draft (m))
  Input Processing/2(CG corrected for payload (m)) -> Terminator/1
  Initial Condition/1(IC) -> 6DOF (In CO)/3(IC)
  Output Processing/1(VesselStates) -> VesselStates/1
  Bus Element In1/1 -> Thrust/2("Gravity (m/s2) ")
  Bus Element In4/1 -> Input Processing/5(Current Speed (m/s))
  Bus Element In/1 -> Input Processing/1(Payload Mass (kg))
  Bus Element In6/1 -> Input Processing/2(Payload Location (m))
  6DOF (In CO)/13(Acc X (m/s2)) -> Bus Creator/13  "Acc_X"
  6DOF (In CO)/14(Acc Y (m/s2)) -> Bus Creator/14  "Acc_Y"
  6DOF (In CO)/15(Acc Z (m/s2)) -> Bus Creator/15  "Acc_Z"
  6DOF (In CO)/16(Angular Acc X (rad/s2)) -> Bus Creator/16  "AngularAcc_X"
  6DOF (In CO)/17(Angular Acc Y (rad/s2)) -> Bus Creator/17  "AngularAcc_Y"
  6DOF (In CO)/18(Angular Acc Z (rad/s2)) -> Bus Creator/18  "AngularAcc_Z"
  [nu_r] -> Hydrodynamics/1(Relative Velocity)
  [H] -> Hydrodynamics/2(Transform CG to CO)
  [Ig] -> Hydrodynamics/3(Inertial Matrix (hull and payload) in CO)
  [X] -> Hydrodynamics/4(X)
  [MA] -> Hydrodynamics/5(Added Mass (Hydrodynamics))
  [Inertials] -> Hydrodynamics/6(Inertials)
  [w3w4w5] -> Hydrodynamics/7(Natural Frequencies)
  Bus Element In2/1 -> Hydrodynamics/8("Gravity (m/s2) ")
  Hydrodynamics/1(Hydrodynamics) -> Sum of Forces and Moments/3(Hydrodynamics)
  Hydrostatic/1(Hydrostatic) -> Sum of Forces and Moments/4(Hydrostatic)
  Inertials/1(Inertials) -> 6DOF (In CO)/2(Inertials)
  Initial Condition1/1(IC) -> Output Processing/2(IC)

== system ROS2_simulink_UE5_0821/Subsystem/Environment                      /Current ==
  Current direction (deg) : Constant  Value=45
  Current speed (m/s) : Constant  Value=0
  Degrees to Radians : simulink_extras/Transformations/Degrees to Radians
  Bus Element Out : Outport  PortName=Current  Element=Current speed (m/s)
  Bus Element Out1 : Outport  PortName=Current  Element=Current direction (rad)
  wires:
  Current direction (deg)/1 -> Degrees to Radians/1
  Degrees to Radians/1 -> Bus Element Out1/1
  Current speed (m/s)/1 -> Bus Element Out/1

== system ROS2_simulink_UE5_0821/Subsystem/Environment                      /Earth ==
  Gravity (m/s2) : Constant  Value=9.81
  Bus Element Out : Outport  PortName=Earth  Element=Gravity (m/s2)
  wires:
  Gravity (m/s2)/1 -> Bus Element Out/1

== system ROS2_simulink_UE5_0821/Subsystem/Environment                      /Water ==
  Water Density (kg/m3) : Constant  Value=1025
  Bus Element Out : Outport  PortName=Water  Element=Water Density (kg/m3)
  wires:
  Water Density (kg/m3)/1 -> Bus Element Out/1

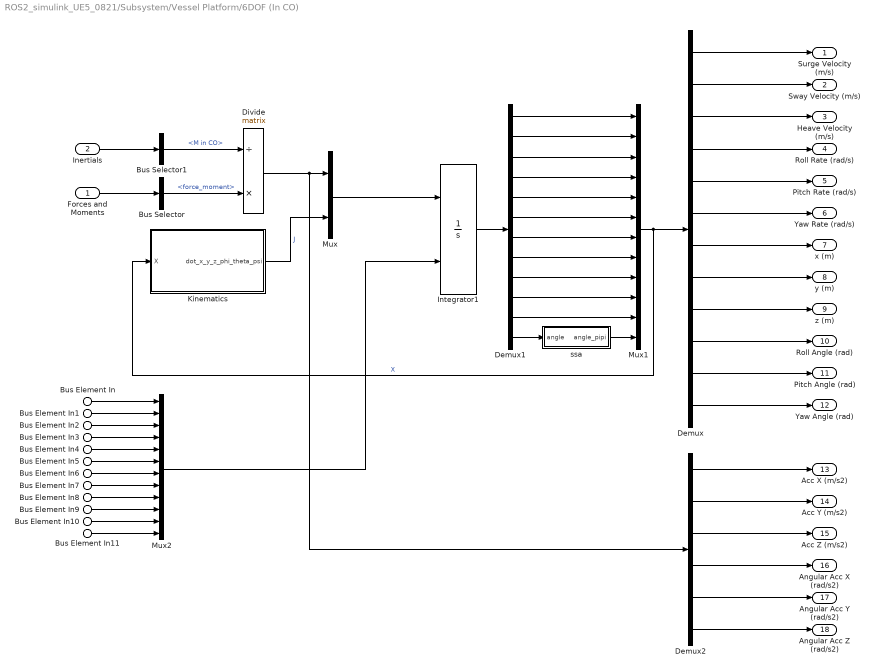
== system ROS2_simulink_UE5_0821/Subsystem/Vessel Platform/6DOF (In CO) ==
  Forces and Moments : Inport
  Inertials : Inport  Port=2
  Bus Element In : Inport  Port=3  PortName=IC  Element=u0_mps
  Bus Element In1 : Inport  Port=3  PortName=IC  Element=v0_mps
  Bus Element In2 : Inport  Port=3  PortName=IC  Element=w0_mps
  Bus Element In3 : Inport  Port=3  PortName=IC  Element=p0_mps
  Bus Element In4 : Inport  Port=3  PortName=IC  Element=q0_mps
  Bus Element In5 : Inport  Port=3  PortName=IC  Element=r0_mps
  Bus Element In6 : Inport  Port=3  PortName=IC  Element=x0_m
  Bus Element In7 : Inport  Port=3  PortName=IC  Element=y0_m
  Bus Element In8 : Inport  Port=3  PortName=IC  Element=z0_m
  Bus Element In9 : Inport  Port=3  PortName=IC  Element=phi0_rad
  Bus Element In10 : Inport  Port=3  PortName=IC  Element=theta0_rad
  Bus Element In11 : Inport  Port=3  PortName=IC  Element=psi0_rad
  Bus Selector : BusSelector  OutputSignals=force_moment
  Bus Selector1 : BusSelector  OutputSignals=M in CO
  Demux : Demux  Outputs=12
  Demux1 : Demux  Outputs=12
  Demux2 : Demux  Outputs=6
  Divide : Product  Inputs=/*  Multiplication=Matrix(*)
  Integrator1 : Integrator  InitialConditionSource=external
  Kinematics : Subsystem
  Mux : Mux  Inputs=2
  Mux1 : Mux  Inputs=12
  Mux2 : Mux  Inputs=12
  "ssa   " : Subsystem
  Surge Velocity (m/s) : Outport
  Sway Velocity (m/s) : Outport  Port=2
  Heave Velocity (m/s) : Outport  Port=3
  Roll Rate (rad/s) : Outport  Port=4
  Pitch Rate (rad/s) : Outport  Port=5
  Yaw Rate (rad/s) : Outport  Port=6
  x (m) : Outport  Port=7
  y (m) : Outport  Port=8
  z (m) : Outport  Port=9
  Roll Angle (rad) : Outport  Port=10
  Pitch Angle (rad) : Outport  Port=11
  Yaw Angle (rad) : Outport  Port=12
  Acc X (m/s2) : Outport  Port=13
  Acc Y (m/s2) : Outport  Port=14
  Acc Z (m/s2) : Outport  Port=15
  Angular Acc X (rad/s2) : Outport  Port=16
  Angular Acc Y (rad/s2) : Outport  Port=17
  Angular Acc Z (rad/s2) : Outport  Port=18
  wires:
  Demux/1 -> Surge Velocity (m/s)/1
  Demux/2 -> Sway Velocity (m/s)/1
  Demux/3 -> Heave Velocity (m/s)/1
  Demux/4 -> Roll Rate (rad/s)/1
  Demux/5 -> Pitch Rate (rad/s)/1
  Demux/6 -> Yaw Rate (rad/s)/1
  Demux/7 -> x (m)/1
  Demux/8 -> y (m)/1
  Demux/9 -> z (m)/1
  Demux/10 -> Roll Angle (rad)/1
  Demux/11 -> Pitch Angle (rad)/1
  Bus Selector1/1 -> Divide/1  "<M in CO>"
  Divide/1 -> Demux2/1, Mux/1
  Forces and Moments/1 -> Bus Selector/1
  Bus Selector/1 -> Divide/2  "<force_moment>"
  Kinematics/1(dot_x_y_z_phi_theta_psi) -> Mux/2  "J"
  Mux/1 -> Integrator1/1
  Demux/12 -> Yaw Angle (rad)/1
  Integrator1/1 -> Demux1/1
  Demux1/1 -> Mux1/1
  Demux1/2 -> Mux1/2
  Demux1/3 -> Mux1/3
  Demux1/4 -> Mux1/4
  Demux1/5 -> Mux1/5
  Demux1/6 -> Mux1/6
  Demux1/7 -> Mux1/7
  Demux1/8 -> Mux1/8
  Demux1/9 -> Mux1/9
  Demux1/10 -> Mux1/10
  Demux1/11 -> Mux1/11
  Demux1/12 -> "ssa   "/1(angle)
  "ssa   "/1(angle_pipi) -> Mux1/12
  Mux1/1 -> Kinematics/1(X), Demux/1  "X"
  Inertials/1 -> Bus Selector1/1
  Mux2/1 -> Integrator1/2
  Bus Element In/1 -> Mux2/1
  Bus Element In1/1 -> Mux2/2
  Bus Element In2/1 -> Mux2/3
  Bus Element In3/1 -> Mux2/4
  Bus Element In4/1 -> Mux2/5
  Bus Element In5/1 -> Mux2/6
  Bus Element In6/1 -> Mux2/7
  Bus Element In7/1 -> Mux2/8
  Bus Element In8/1 -> Mux2/9
  Bus Element In9/1 -> Mux2/10
  Bus Element In10/1 -> Mux2/11
  Bus Element In11/1 -> Mux2/12
  Demux2/1 -> Acc X (m/s2)/1
  Demux2/2 -> Acc Y (m/s2)/1
  Demux2/3 -> Acc Z (m/s2)/1
  Demux2/4 -> Angular Acc X (rad/s2)/1
  Demux2/5 -> Angular Acc Y (rad/s2)/1
  Demux2/6 -> Angular Acc Z (rad/s2)/1

== system ROS2_simulink_UE5_0821/Subsystem/Vessel Platform/Hydrodynamics ==
  Relative Velocity : Inport
  Transform CG to CO : Inport  Port=2
  Inertial Matrix (hull and payload) in CO : Inport  Port=3
  X : Inport  Port=4
  Added Mass (Hydrodynamics) : Inport  Port=5
  Inertials : Inport  Port=6
  Natural Frequencies : Inport  Port=7
  "Gravity (m/s2) " : Inport  Port=8
  "Coriolis " : Subsystem
  Damping (Hydrodynamics) : Subsystem
  "Inertials " : InportShadow  Port=6
  "Relative Velocity " : InportShadow
  Bus Element Out : Outport  PortName=Hydrodynamics  Element=Coriolis
  Bus Element Out1 : Outport  PortName=Hydrodynamics  Element=Damping
  wires:
  Relative Velocity/1 -> "Coriolis "/1(Relative Velocity)
  X/1 -> "Coriolis "/4(X)
  Transform CG to CO/1 -> "Coriolis "/2(Transform CG to CO)
  Inertial Matrix (hull and payload) in CO/1 -> "Coriolis "/3(Inertial Matrix (hull and payload) in CO)
  "Gravity (m/s2) "/1 -> Damping (Hydrodynamics)/4("Gravity (m/s2) ")
  Added Mass (Hydrodynamics)/1 -> "Coriolis "/5(Added Mass (Hydrodynamics))
  Natural Frequencies/1 -> Damping (Hydrodynamics)/3(Natural Frequencies)
  Inertials/1 -> "Coriolis "/6(Inertials)
  "Relative Velocity "/1 -> Damping (Hydrodynamics)/1(Relative Velocity)
  "Inertials "/1 -> Damping (Hydrodynamics)/2(Inertials)
  "Coriolis "/1(Coriolis) -> Bus Element Out/1
  Damping (Hydrodynamics)/1(Damping) -> Bus Element Out1/1

== system ROS2_simulink_UE5_0821/Subsystem/Vessel Platform/Hydrostatic ==
  X : Inport
  G : Inport  Port=2
  Ballast : Subsystem
  Bus Selector : BusSelector  OutputSignals=x_m,y_m,z_m,phi_rad,theta_rad,psi_rad
  Mux2 : Mux  Inputs=6
  Product : Product  Multiplication=Matrix(*)
  Reshape : Reshape  OutputDimensionality=Column vector (2-D)
  Bus Element Out : Outport  PortName=Hydrostatic  Element=Hydrostatic
  Bus Element Out1 : Outport  PortName=Hydrostatic  Element=Ballast
  wires:
  Mux2/1 -> Reshape/1
  G/1 -> Product/1
  Reshape/1 -> Product/2  "eta"
  X/1 -> Bus Selector/1
  Bus Selector/1 -> Mux2/1  "<x_m>"
  Bus Selector/2 -> Mux2/2  "<y_m>"
  Bus Selector/3 -> Mux2/3  "<z_m>"
  Bus Selector/4 -> Mux2/4  "<phi_rad>"
  Bus Selector/5 -> Mux2/5  "<theta_rad>"
  Bus Selector/6 -> Mux2/6  "<psi_rad>"
  Product/1 -> Bus Element Out/1
  Ballast/1(Ballast) -> Bus Element Out1/1

== system ROS2_simulink_UE5_0821/Subsystem/Vessel Platform/Inertials ==
  Inertials : Outport
  wires:
  [Inertials] -> Inertials/1

== system ROS2_simulink_UE5_0821/Subsystem/Vessel Platform/Initial Condition ==
  Demux : Demux  Outputs=14
  Initial States : Constant  Value=[IC.u_mps IC.v_mps IC.w_mps IC.p_rps IC.q_rps IC.r_rps IC.x_m IC.y_m IC.z_m IC.phi_rad IC.theta_rad IC.psi_rad IC.latitude_deg IC.longitude_deg]
  Bus Element Out : Outport  PortName=IC  Element=u0_mps
  Bus Element Out1 : Outport  PortName=IC  Element=v0_mps
  Bus Element Out2 : Outport  PortName=IC  Element=w0_mps
  Bus Element Out3 : Outport  PortName=IC  Element=p0_mps
  Bus Element Out4 : Outport  PortName=IC  Element=q0_mps
  Bus Element Out5 : Outport  PortName=IC  Element=r0_mps
  Bus Element Out6 : Outport  PortName=IC  Element=x0_m
  Bus Element Out7 : Outport  PortName=IC  Element=y0_m
  Bus Element Out8 : Outport  PortName=IC  Element=z0_m
  Bus Element Out9 : Outport  PortName=IC  Element=phi0_rad
  Bus Element Out10 : Outport  PortName=IC  Element=theta0_rad
  Bus Element Out11 : Outport  PortName=IC  Element=psi0_rad
  Bus Element Out12 : Outport  PortName=IC  Element=latitude0_deg
  Bus Element Out13 : Outport  PortName=IC  Element=longitude0_deg
  wires:
  Initial States/1 -> Demux/1
  Demux/1 -> Bus Element Out/1  "u0_mps"
  Demux/2 -> Bus Element Out1/1  "v0_mps"
  Demux/3 -> Bus Element Out2/1  "w0_mps"
  Demux/4 -> Bus Element Out3/1  "p0_mps"
  Demux/5 -> Bus Element Out4/1  "q0_mps"
  Demux/6 -> Bus Element Out5/1  "r0_mps"
  Demux/7 -> Bus Element Out6/1  "x0_m"
  Demux/8 -> Bus Element Out7/1  "y0_m"
  Demux/9 -> Bus Element Out8/1  "z0_m"
  Demux/10 -> Bus Element Out9/1  "phi0_rad"
  Demux/11 -> Bus Element Out10/1  "theta0_rad"
  Demux/12 -> Bus Element Out11/1  "psi0_rad"
  Demux/13 -> Bus Element Out12/1  "latitude0_deg"
  Demux/14 -> Bus Element Out13/1  "longitude0_deg"

== system ROS2_simulink_UE5_0821/Subsystem/Vessel Platform/Initial Condition1 ==
  Demux : Demux  Outputs=14
  Initial States : Constant  Value=[IC.u_mps IC.v_mps IC.w_mps IC.p_rps IC.q_rps IC.r_rps IC.x_m IC.y_m IC.z_m IC.phi_rad IC.theta_rad IC.psi_rad IC.latitude_deg IC.longitude_deg]
  Bus Element Out : Outport  PortName=IC  Element=u0_mps
  Bus Element Out1 : Outport  PortName=IC  Element=v0_mps
  Bus Element Out2 : Outport  PortName=IC  Element=w0_mps
  Bus Element Out3 : Outport  PortName=IC  Element=p0_mps
  Bus Element Out4 : Outport  PortName=IC  Element=q0_mps
  Bus Element Out5 : Outport  PortName=IC  Element=r0_mps
  Bus Element Out6 : Outport  PortName=IC  Element=x0_m
  Bus Element Out7 : Outport  PortName=IC  Element=y0_m
  Bus Element Out8 : Outport  PortName=IC  Element=z0_m
  Bus Element Out9 : Outport  PortName=IC  Element=phi0_rad
  Bus Element Out10 : Outport  PortName=IC  Element=theta0_rad
  Bus Element Out11 : Outport  PortName=IC  Element=psi0_rad
  Bus Element Out12 : Outport  PortName=IC  Element=latitude0_deg
  Bus Element Out13 : Outport  PortName=IC  Element=longitude0_deg
  wires:
  Initial States/1 -> Demux/1
  Demux/1 -> Bus Element Out/1  "u0_mps"
  Demux/2 -> Bus Element Out1/1  "v0_mps"
  Demux/3 -> Bus Element Out2/1  "w0_mps"
  Demux/4 -> Bus Element Out3/1  "p0_mps"
  Demux/5 -> Bus Element Out4/1  "q0_mps"
  Demux/6 -> Bus Element Out5/1  "r0_mps"
  Demux/7 -> Bus Element Out6/1  "x0_m"
  Demux/8 -> Bus Element Out7/1  "y0_m"
  Demux/9 -> Bus Element Out8/1  "z0_m"
  Demux/10 -> Bus Element Out9/1  "phi0_rad"
  Demux/11 -> Bus Element Out10/1  "theta0_rad"
  Demux/12 -> Bus Element Out11/1  "psi0_rad"
  Demux/13 -> Bus Element Out12/1  "latitude0_deg"
  Demux/14 -> Bus Element Out13/1  "longitude0_deg"

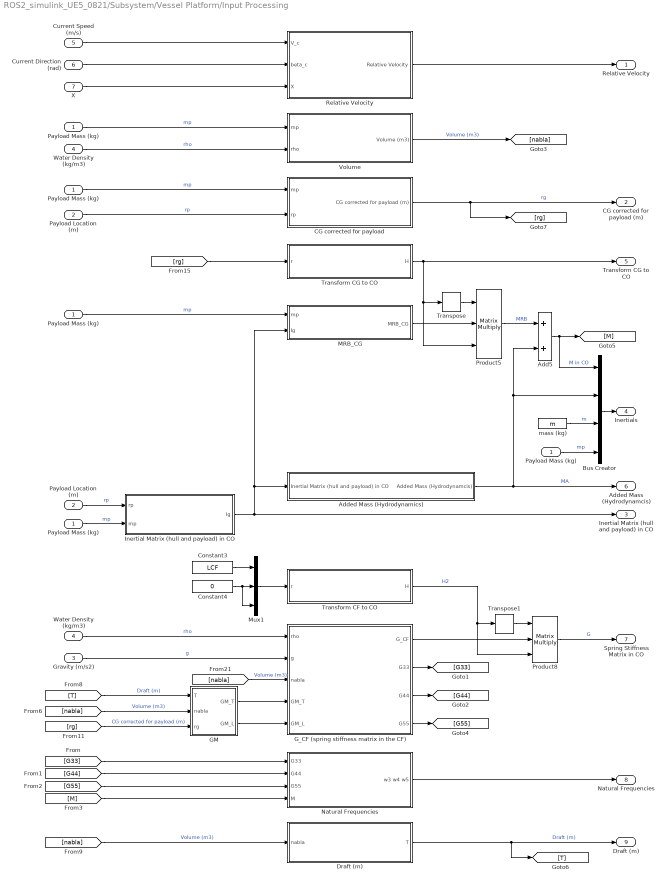
== system ROS2_simulink_UE5_0821/Subsystem/Vessel Platform/Input Processing ==
  Payload Mass (kg) : Inport
  Payload Location (m) : Inport  Port=2
  Gravity (m/s2) : Inport  Port=3
  Water Density (kg/m3) : Inport  Port=4
  Current Speed (m/s) : Inport  Port=5
  Current Direction (rad) : Inport  Port=6
  X : Inport  Port=7
  "  Payload Mass (kg)  " : InportShadow
  " Payload Mass (kg) " : InportShadow
  " mass (kg) " : Constant  Value=m
  Add5 : Sum
  "Added Mass (Hydrodynamics) " : Subsystem
  Bus Creator : BusCreator  Inputs=4
  CG corrected for payload : Subsystem
  Constant3 : Constant  Value=LCF
  Constant4 : Constant  Value=0
  "Draft (m) " : Subsystem
  GM : Subsystem
  G_CF (spring stiffness matrix in the CF) : Subsystem
  "Inertial Matrix (hull and payload) in CO " : Subsystem
  MRB_CG : Subsystem
  Mux1 : Mux  Inputs=3
  "Natural Frequencies " : Subsystem
  "Payload Location (m) " : InportShadow  Port=2
  "Payload Mass (kg) " : InportShadow
  "Payload Mass (kg)  " : InportShadow
  Product5 : Product  Inputs=3  Multiplication=Matrix(*)
  Product8 : Product  Inputs=3  Multiplication=Matrix(*)
  "Relative Velocity " : Subsystem
  Transform CF to CO : Subsystem
  "Transform CG to CO " : Subsystem
  Transpose : matrix_library/Transpose
  Transpose1 : matrix_library/Transpose
  Volume : Subsystem
  "Water Density (kg/m3) " : InportShadow  Port=4
  Relative Velocity : Outport
  CG corrected for payload (m) : Outport  Port=2
  Inertial Matrix (hull and payload) in CO : Outport  Port=3
  Inertials : Outport  Port=4
  Transform CG to CO : Outport  Port=5
  Added Mass (Hydrodynamcis) : Outport  Port=6
  Spring Stiffness Matrix in CO : Outport  Port=7
  Natural Frequencies : Outport  Port=8
  Draft (m) : Outport  Port=9
  wires:
  "Transform CG to CO "/1(H) -> Transform CG to CO/1, Transpose/1, Product5/3
  Transpose/1 -> Product5/1
  Product5/1 -> Add5/1  "MRB"
  Current Speed (m/s)/1 -> "Relative Velocity "/1(V_c)
  "Relative Velocity "/1(Relative Velocity) -> Relative Velocity/1
  Current Direction (rad)/1 -> "Relative Velocity "/2(beta_c)
  X/1 -> "Relative Velocity "/3(X)
  "Added Mass (Hydrodynamics) "/1(Added Mass (Hydrodynamcis)) -> Add5/2, Bus Creator/2, Added Mass (Hydrodynamcis)/1  "MA"
  Add5/1 -> [M], Bus Creator/1  "M in CO"
  Bus Creator/1 -> Inertials/1
  Constant3/1 -> Mux1/1
  Constant4/1 -> Mux1/3, Mux1/2
  Mux1/1 -> Transform CF to CO/1(r)
  Transform CF to CO/1(H) -> Product8/3, Transpose1/1  "H2"
  Transpose1/1 -> Product8/1
  Product8/1 -> Spring Stiffness Matrix in CO/1  "G"
  " mass (kg) "/1 -> Bus Creator/3  "m"
  "Payload Mass (kg)  "/1 -> Bus Creator/4  "mp"
  Payload Mass (kg)/1 -> Volume/1(mp)  "mp"
  Water Density (kg/m3)/1 -> Volume/2(rho)  "rho"
  Volume/1(Volume (m3)) -> [nabla]  "Volume (m3)"
  CG corrected for payload/1(CG corrected for payload (m)) -> [rg], CG corrected for payload (m)/1  "rg"
  "Payload Mass (kg) "/1 -> CG corrected for payload/1(mp)  "mp"
  Payload Location (m)/1 -> CG corrected for payload/2(rp)  "rp"
  " Payload Mass (kg) "/1 -> MRB_CG/1(mp)  "mp"
  MRB_CG/1(MRB_CG) -> Product5/2
  [rg] -> "Transform CG to CO "/1(r)
  "Inertial Matrix (hull and payload) in CO "/1(Ig) -> Inertial Matrix (hull and payload) in CO/1, MRB_CG/2(Ig), "Added Mass (Hydrodynamics) "/1(Inertial Matrix (hull and payload) in CO)
  "Payload Location (m) "/1 -> "Inertial Matrix (hull and payload) in CO "/1(rp)  "rp"
  "  Payload Mass (kg)  "/1 -> "Inertial Matrix (hull and payload) in CO "/2(mp)  "mp"
  "Water Density (kg/m3) "/1 -> G_CF (spring stiffness matrix in the CF)/1(rho)  "rho"
  Gravity (m/s2)/1 -> G_CF (spring stiffness matrix in the CF)/2(g)  "g"
  [nabla] -> G_CF (spring stiffness matrix in the CF)/3(nabla)  "Volume (m3)"
  G_CF (spring stiffness matrix in the CF)/1(G_CF) -> Product8/2
  G_CF (spring stiffness matrix in the CF)/2(G33) -> [G33]
  G_CF (spring stiffness matrix in the CF)/3(G44) -> [G44]
  G_CF (spring stiffness matrix in the CF)/4(G55) -> [G55]
  GM/2(GM_L) -> G_CF (spring stiffness matrix in the CF)/5(GM_L)
  GM/1(GM_T) -> G_CF (spring stiffness matrix in the CF)/4(GM_T)
  [G33] -> "Natural Frequencies "/1(G33)
  [M] -> "Natural Frequencies "/4(M)
  [G44] -> "Natural Frequencies "/2(G44)
  [G55] -> "Natural Frequencies "/3(G55)
  "Natural Frequencies "/1(w3 w4 w5) -> Natural Frequencies/1
  [nabla] -> "Draft (m) "/1(nabla)  "Volume (m3)"
  "Draft (m) "/1(T) -> [T], Draft (m)/1  "Draft (m)"
  [T] -> GM/1(T)  "Draft (m)"
  [rg] -> GM/3(rg)  "CG corrected for payload (m)"
  [nabla] -> GM/2(nabla)  "Volume (m3)"
